simulink model "linear_system"  (R2023b)
settings: Solver=VariableStepAuto  StartTime=0.0  StopTime=60  RelTol=1e-3
values from neighbouring files (symbols this model uses):
  Alin = [0    -k/Jl + m*g*l*sin(x2_bar)/Jl                     0           k/Jl ... (first row only)    [collaborative_class_main.m]    (also in n0_collaborative_class_main.m = [ 0           -k/Jl + m*g*l*sin(x2_bar)/Jl             0    )
  Blin = [0; 0; 1/Jm; 0]    [collaborative_class_main.m]    (also in n0_collaborative_class_main.m)
  K = place(Alin, Blin, p)    [collaborative_class_main.m]    (also in n0_collaborative_class_main.m)
  K_H2_V = K_H2(:, 5)    [collaborative_class_main.m]    (also in n0_collaborative_class_main.m)
  K_H2_X = K_H2(:,1:4)    [collaborative_class_main.m]    (also in n0_collaborative_class_main.m)
  K_lq = R^(-1)*Blin'*P_lq    [n0_collaborative_class_main.m]
  K_lqeta = K_lqe(:, 5)    [collaborative_class_main.m]    (also in n0_collaborative_class_main.m = K_lq_ext(:,5))
  K_lqx = K_lqe(:,1:4)    [collaborative_class_main.m]    (also in n0_collaborative_class_main.m = K_lq_ext(:,1:4))
  Kv = -K_ext(1, 5)    [collaborative_class_main.m]    (also in n0_collaborative_class_main.m)
  Kx = -K_ext(1, 1:4)    [collaborative_class_main.m]    (also in n0_collaborative_class_main.m)
  x_bar = [x1_bar x2_bar x3_bar x4_bar]    [collaborative_class_main.m]    (also in n0_collaborative_class_main.m; svc_robot.m = [x1_bar x2_bar x3_bar x4_bar]')
settings Model: Creator=teoma  LastModifiedBy=alexandraspertini

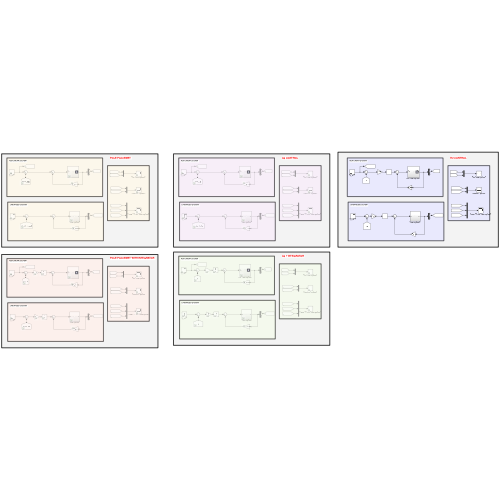
[thumbnail: Simulink's stored preview of the top-level diagram]
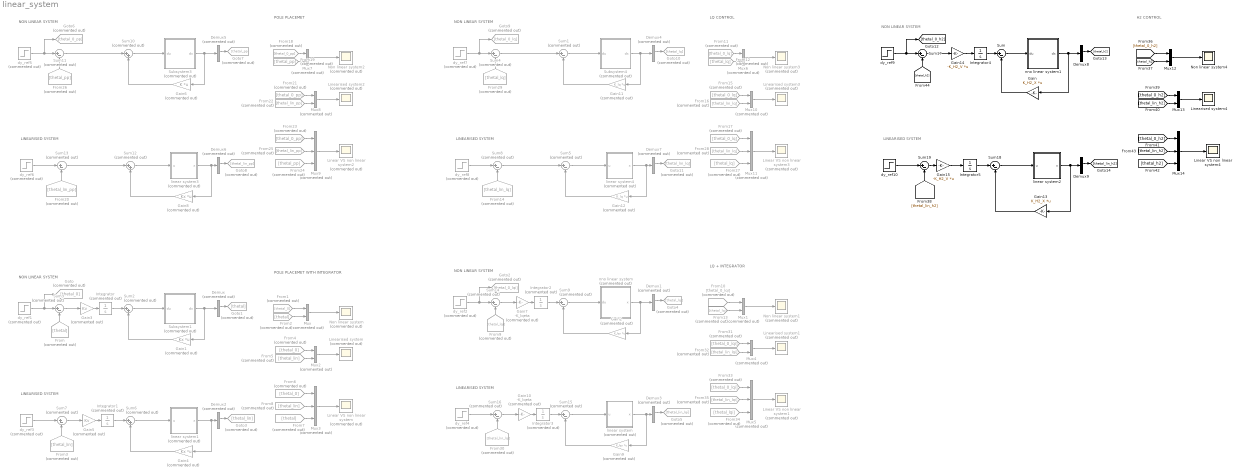
== system linear_system ==
  note: POLE PLACEMET WITH INTEGRATOR
  note: NON LINEAR SYSTEM
  note: LINEARISED SYSTEM
  note: POLE PLACEMET
  note: LINEARISED SYSTEM
  note: NON LINEAR SYSTEM
  note: NON LINEAR SYSTEM
  note: LQ CONTROL
  note: LINEARISED SYSTEM
  note: NON LINEAR SYSTEM
  note: LINEARISED SYSTEM
  note: LQ + INTEGRATOR
  note: LINEARISED SYSTEM
  note: H2 CONTROL
  note: NON LINEAR SYSTEM
  Demux{,1..7} (8 alike) : Demux  Commented=on
  Demux8 : Demux
  Demux9 : Demux
  From : From  Commented=on  GotoTag=thetal
  From1 : From  Commented=on  GotoTag=thetal_0
  From10 : From  Commented=on  GotoTag=thetal_0_lqi
  From11 : From  Commented=on  GotoTag=thetal_0_lq
  From12 : From  Commented=on  GotoTag=thetal_lq
  From13 : From  Commented=on  GotoTag=thetal_lqi
  From14 : From  Commented=on  GotoTag=thetal_lin_lq
  From15 : From  Commented=on  GotoTag=thetal_0_lq
  From16 : From  Commented=on  GotoTag=thetal_lin_lq
  From17 : From  Commented=on  GotoTag=thetal_0_lq
  From18 : From  Commented=on  GotoTag=thetal_0_pp
  From19 : From  Commented=on  GotoTag=thetal_pp
  From2 : From  Commented=on  GotoTag=thetal
  From20 : From  Commented=on  GotoTag=thetal_lin_pp
  From21 : From  Commented=on  GotoTag=thetal_0_pp
  From22 : From  Commented=on  GotoTag=thetal_lin_pp
  From23 : From  Commented=on  GotoTag=thetal_0_pp
  From24 : From  Commented=on  GotoTag=thetal_pp
  From25 : From  Commented=on  GotoTag=thetal_lin_pp
  From26 : From  Commented=on  GotoTag=thetal_pp
  From27 : From  Commented=on  GotoTag=thetal_lq
  From28 : From  Commented=on  GotoTag=thetal_lin_lq
  From29 : From  Commented=on  GotoTag=thetal_lq
  From3 : From  Commented=on  GotoTag=thetal_lin
  From30 : From  Commented=on  GotoTag=thetal_lin_lqi
  From31 : From  Commented=on  GotoTag=thetal_0_lqi
  From32 : From  Commented=on  GotoTag=thetal_lin_lqi
  From33 : From  Commented=on  GotoTag=thetal_0_lqi
  From34 : From  Commented=on  GotoTag=thetal_lqi
  From35 : From  Commented=on  GotoTag=thetal_lin_lqi
  From4 : From  Commented=on  GotoTag=thetal_0
  From5 : From  Commented=on  GotoTag=thetal_lin
  From6 : From  Commented=on  GotoTag=thetal_0
  From7 : From  Commented=on  GotoTag=thetal
  From8 : From  Commented=on  GotoTag=thetal_lin
  From9 : From  Commented=on  GotoTag=thetal_lqi
  Gain : Gain  Gain=K_H2_X  Multiplication=Matrix(K*u) (u vector)
  Gain1 : Gain  Commented=on  Gain=Kx  Multiplication=Matrix(K*u) (u vector)
  Gain10 : Gain  Commented=on  Gain=-K_lqeta
  Gain11 : Gain  Commented=on  Gain=K_lq  Multiplication=Matrix(K*u) (u vector)
  Gain12 : Gain  Commented=on  Gain=K_lq  Multiplication=Matrix(K*u) (u vector)
  Gain13 : Gain  Gain=K_H2_X  Multiplication=Matrix(K*u) (u vector)
  Gain14 : Gain  Gain=-K_H2_V  Multiplication=Matrix(K*u) (u vector)
  Gain15 : Gain  Gain=-K_H2_V  Multiplication=Matrix(K*u) (u vector)
  Gain2 : Gain  Commented=on  Gain=K_lqx  Multiplication=Matrix(K*u) (u vector)
  Gain3 : Gain  Commented=on  Gain=Kv
  Gain4 : Gain  Commented=on  Gain=Kx  Multiplication=Matrix(K*u) (u vector)
  Gain5 : Gain  Commented=on  Gain=Kv
  Gain6 : Gain  Commented=on  Gain=K  Multiplication=Matrix(K*u) (u vector)
  Gain7 : Gain  Commented=on  Gain=-K_lqeta
  Gain8 : Gain  Commented=on  Gain=Kx  Multiplication=Matrix(K*u) (u vector)
  Gain9 : Gain  Commented=on  Gain=K_lqx  Multiplication=Matrix(K*u) (u vector)
  Goto : Goto  Commented=on  GotoTag=thetal_0
  Goto1 : Goto  Commented=on  GotoTag=thetal
  Goto10 : Goto  Commented=on  GotoTag=thetal_lq
  Goto11 : Goto  Commented=on  GotoTag=thetal_lin_lq
  Goto2 : Goto  Commented=on  GotoTag=thetal_0_lqi
  Goto3 : Goto  Commented=on  GotoTag=thetal_lin
  Goto4 : Goto  Commented=on  GotoTag=thetal_lqi
  Goto5 : Goto  Commented=on  GotoTag=thetal_lin_lqi
  Goto6 : Goto  Commented=on  GotoTag=thetal_0_pp
  Goto7 : Goto  Commented=on  GotoTag=thetal_pp
  Goto8 : Goto  Commented=on  GotoTag=thetal_lin_pp
  Goto9 : Goto  Commented=on  GotoTag=thetal_0_lq
  Integrator{,1..3} (4 alike) : Integrator  Commented=on
  Integrator4 : Integrator
  Integrator5 : Integrator
  Linear VS non linear system{,1..3} (4 alike) : Scope  Commented=on
  Linear VS non linear system4 : Scope
  Linearised system{,1..3} (4 alike) : Scope  Commented=on
  Linearised system4 : Scope
  Mux{,1..2,4,6..8,10} (8 alike) : Mux  Commented=on  Inputs=2
  Mux{3,5,9,11} (4 alike) : Mux  Commented=on  Inputs=3
  Mux12 : Mux  Inputs=2
  Mux13 : Mux  Inputs=2
  Mux14 : Mux  Inputs=3
  Non linear system{,1..3} (4 alike) : Scope  Commented=on
  Non linear system4 : Scope
  Subsystem1 : Subsystem  Commented=on
  Subsystem3 : Subsystem  Commented=on
  Subsystem4 : Subsystem  Commented=on
  Sum{,17..19} (4 alike) : Sum  Inputs=|+-
  Sum{1,3..5,7..9,11,13..16} (12 alike) : Sum  Commented=on  Inputs=|+-
  Sum{2,6,10,12} (4 alike) : Sum  Commented=on  Inputs=|++
  dy_ref{1,3,5..6} (4 alike) : Step  Commented=on  After=pi/24  SampleTime=0
  dy_ref10 : Step  Time=0  After=pi/36  SampleTime=0
  dy_ref2 : Step  Commented=on  Time=0  After=pi/36  SampleTime=0
  dy_ref4 : Step  Commented=on  Time=0  After=pi/36  SampleTime=0
  dy_ref7 : Step  Commented=on  After=pi/36  SampleTime=0
  dy_ref8 : Step  Commented=on  After=pi/36  SampleTime=0
  dy_ref9 : Step  Time=0  After=pi/36  SampleTime=0
  linear system : Subsystem  Commented=on
  linear system1 : Subsystem  Commented=on
  linear system2 : Subsystem
  linear system3 : Subsystem  Commented=on
  linear system4 : Subsystem  Commented=on
  nno linear system : Subsystem  Commented=on
  nno linear system1 : Subsystem
  wires:
  Subsystem1/1(dx) -> Gain1/1, Demux/1
  Sum2/1 -> Subsystem1/1(du)
  Gain1/1 -> Sum2/2
  dy_ref1/1 -> Goto/1, Sum3/1
  Mux/1 -> Non linear system/1
  Sum3/1 -> Gain3/1
  Gain3/1 -> Integrator/1
  Integrator/1 -> Sum2/1
  Demux/2 -> Goto1/1
  From/1 -> Sum3/2
  From1/1 -> Mux/1
  From2/1 -> Mux/2
  dy_ref3/1 -> Sum7/1
  Sum7/1 -> Gain5/1
  Sum6/1 -> linear system1/1(u)
  From5/1 -> Mux2/2
  Gain4/1 -> Sum6/2
  Mux2/1 -> Linearised system/1
  Gain5/1 -> Integrator1/1
  Integrator1/1 -> Sum6/1
  From4/1 -> Mux2/1
  From3/1 -> Sum7/2
  Demux2/2 -> Goto3/1
  linear system1/1(x) -> Gain4/1, Demux2/1
  From6/1 -> Mux3/1
  From7/1 -> Mux3/3
  From8/1 -> Mux3/2
  Mux3/1 -> Linear VS non linear system/1
  Sum10/1 -> Subsystem3/1(du)
  Mux7/1 -> Non linear system2/1
  From21/1 -> Mux8/1
  From19/1 -> Mux7/2
  Gain6/1 -> Sum10/2
  Subsystem3/1(dx) -> Gain6/1, Demux5/1
  From23/1 -> Mux9/1
  Mux8/1 -> Linearised system2/1
  linear system3/1(x) -> Gain8/1, Demux6/1
  Demux5/2 -> Goto7/1
  From26/1 -> Sum11/2
  From18/1 -> Mux7/1
  Gain8/1 -> Sum12/2
  Demux6/2 -> Goto8/1
  From20/1 -> Sum13/2
  Mux9/1 -> Linear VS non linear system2/1
  dy_ref6/1 -> Sum13/1
  From22/1 -> Mux8/2
  From25/1 -> Mux9/2
  Sum12/1 -> linear system3/1(u)
  From24/1 -> Mux9/3
  dy_ref5/1 -> Goto6/1, Sum11/1
  Sum11/1 -> Sum10/1
  Sum13/1 -> Sum12/1
  From33/1 -> Mux5/1
  Sum8/1 -> Sum5/1
  From29/1 -> Sum4/2
  Subsystem4/1(dx) -> Gain11/1, Demux4/1
  Integrator3/1 -> Sum15/1
  From17/1 -> Mux11/1
  Sum1/1 -> Subsystem4/1(du)
  Mux1/1 -> Non linear system1/1
  From32/1 -> Mux4/2
  Mux10/1 -> Linearised system3/1
  Demux3/2 -> Goto5/1
  Demux7/2 -> Goto11/1
  From15/1 -> Mux10/1
  Demux1/2 -> Goto4/1
  Mux6/1 -> Non linear system3/1
  From14/1 -> Sum8/2
  From11/1 -> Mux6/1
  From27/1 -> Mux11/3
  Sum4/1 -> Sum1/1
  From31/1 -> Mux4/1
  Gain11/1 -> Sum1/2
  Sum15/1 -> linear system/1(u)
  dy_ref2/1 -> Goto2/1, Sum14/1
  Gain7/1 -> Integrator2/1
  Gain2/1 -> Sum9/2
  From10/1 -> Mux1/1
  From12/1 -> Mux6/2
  Gain9/1 -> Sum15/2
  dy_ref4/1 -> Sum16/1
  nno linear system/1(x) -> Gain2/1, Demux1/1
  From35/1 -> Mux5/2
  Gain10/1 -> Integrator3/1
  Sum16/1 -> Gain10/1
  Sum5/1 -> linear system4/1(u)
  From9/1 -> Sum14/2
  dy_ref8/1 -> Sum8/1
  From13/1 -> Mux1/2
  linear system/1(x) -> Gain9/1, Demux3/1
  Sum14/1 -> Gain7/1
  dy_ref7/1 -> Goto9/1, Sum4/1
  Mux4/1 -> Linearised system1/1
  Mux11/1 -> Linear VS non linear system3/1
  linear system4/1(x) -> Gain12/1, Demux7/1
  From16/1 -> Mux10/2
  From28/1 -> Mux11/2
  Sum9/1 -> nno linear system/1(du)
  Mux5/1 -> Linear VS non linear system1/1
  Demux4/2 -> Goto10/1
  From30/1 -> Sum16/2
  Gain12/1 -> Sum5/2
  From34/1 -> Mux5/3
  Integrator2/1 -> Sum9/1
  [thetal_lin_h2] -> Mux13/2
  Demux9/2 -> [thetal_lin_h2]
  [thetal_lin_h2] -> Mux14/2
  [thetal_lin_h2] -> Sum19/2
  [thetal_h2] -> Mux12/2
  Mux12/1 -> Non linear system4/1
  [thetal_h2] -> Sum17/2
  [thetal_h2] -> Mux14/3
  dy_ref10/1 -> Sum19/1
  [thetal_0_h2] -> Mux12/1
  Demux8/2 -> [thetal_h2]
  [thetal_0_h2] -> Mux13/1
  nno linear system1/1(dx) -> Gain/1, Demux8/1
  dy_ref9/1 -> [thetal_0_h2], Sum17/1
  [thetal_0_h2] -> Mux14/1
  Mux14/1 -> Linear VS non linear system4/1
  linear system2/1(x) -> Gain13/1, Demux9/1
  Mux13/1 -> Linearised system4/1
  Gain/1 -> Sum/2
  Sum/1 -> nno linear system1/1(du)
  Sum18/1 -> linear system2/1(u)
  Gain13/1 -> Sum18/2
  Gain14/1 -> Integrator4/1
  Gain15/1 -> Integrator5/1
  Sum17/1 -> Gain14/1
  Integrator4/1 -> Sum/1
  Sum19/1 -> Gain15/1
  Integrator5/1 -> Sum18/1

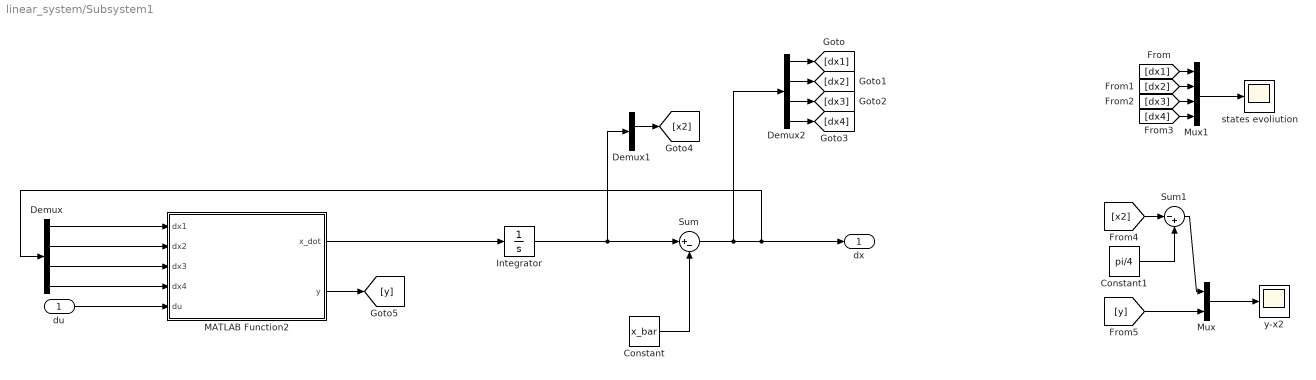
== system linear_system/Subsystem1 ==
  du : Inport
  Constant : Constant  Value=x_bar
  Constant1 : Constant  Value=pi/4
  Demux : Demux
  Demux1 : Demux
  Demux2 : Demux
  Integrator : Integrator  InitialCondition=0.001
  MATLAB Function2 : MATLAB Function  TreatAsAtomicUnit=on
  Mux : Mux  Inputs=2
  Mux1 : Mux
  Sum : Sum  Inputs=|+-
  Sum1 : Sum  Inputs=|-+
  "states evoliution " : Scope
  y-x2 : Scope
  dx : Outport
  wires:
  du/1 -> MATLAB Function2/5(du)
  MATLAB Function2/2(y) -> [y]
  Demux/1 -> MATLAB Function2/1(dx1)
  Demux/2 -> MATLAB Function2/2(dx2)
  Demux/3 -> MATLAB Function2/3(dx3)
  Demux/4 -> MATLAB Function2/4(dx4)
  Constant/1 -> Sum/2
  MATLAB Function2/1(x_dot) -> Integrator/1
  Integrator/1 -> Demux1/1, Sum/1
  Sum/1 -> Demux2/1, dx/1, Demux/1
  Mux/1 -> y-x2/1
  Sum1/1 -> Mux/1
  Constant1/1 -> Sum1/2
  Demux2/1 -> [dx1]
  Demux2/2 -> [dx2]
  Demux2/3 -> [dx3]
  Demux2/4 -> [dx4]
  [dx1] -> Mux1/1
  [dx2] -> Mux1/2
  [dx3] -> Mux1/3
  [dx4] -> Mux1/4
  Mux1/1 -> "states evoliution "/1
  Demux1/2 -> [x2]
  [x2] -> Sum1/1
  [y] -> Mux/2

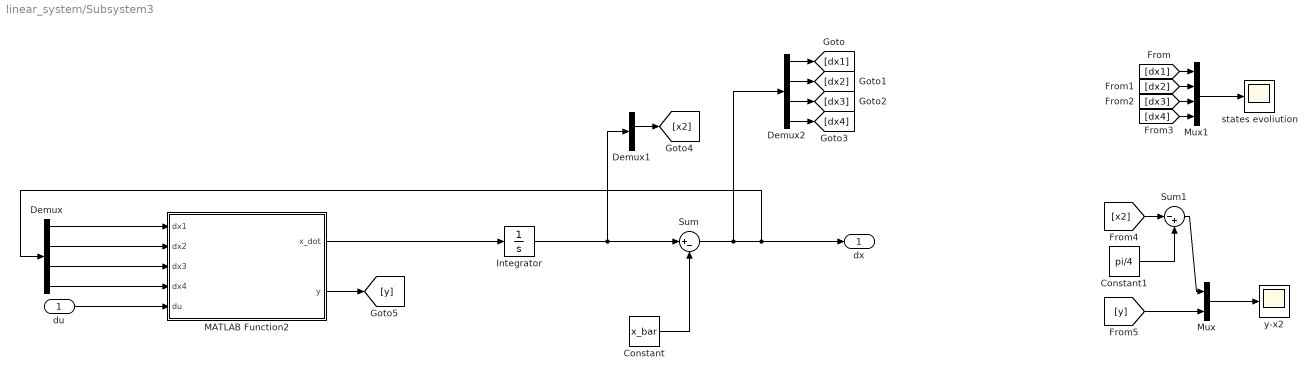
== system linear_system/Subsystem3 ==
  du : Inport
  Constant : Constant  Value=x_bar
  Constant1 : Constant  Value=pi/4
  Demux : Demux
  Demux1 : Demux
  Demux2 : Demux
  Integrator : Integrator  InitialCondition=0.001
  MATLAB Function2 : MATLAB Function  TreatAsAtomicUnit=on
  Mux : Mux  Inputs=2
  Mux1 : Mux
  Sum : Sum  Inputs=|+-
  Sum1 : Sum  Inputs=|-+
  "states evoliution " : Scope
  y-x2 : Scope
  dx : Outport
  wires:
  du/1 -> MATLAB Function2/5(du)
  MATLAB Function2/2(y) -> [y]
  Demux/1 -> MATLAB Function2/1(dx1)
  Demux/2 -> MATLAB Function2/2(dx2)
  Demux/3 -> MATLAB Function2/3(dx3)
  Demux/4 -> MATLAB Function2/4(dx4)
  Constant/1 -> Sum/2
  MATLAB Function2/1(x_dot) -> Integrator/1
  Integrator/1 -> Demux1/1, Sum/1
  Sum/1 -> Demux2/1, dx/1, Demux/1
  Mux/1 -> y-x2/1
  Sum1/1 -> Mux/1
  Constant1/1 -> Sum1/2
  Demux2/1 -> [dx1]
  Demux2/2 -> [dx2]
  Demux2/3 -> [dx3]
  Demux2/4 -> [dx4]
  [dx1] -> Mux1/1
  [dx2] -> Mux1/2
  [dx3] -> Mux1/3
  [dx4] -> Mux1/4
  Mux1/1 -> "states evoliution "/1
  Demux1/2 -> [x2]
  [x2] -> Sum1/1
  [y] -> Mux/2

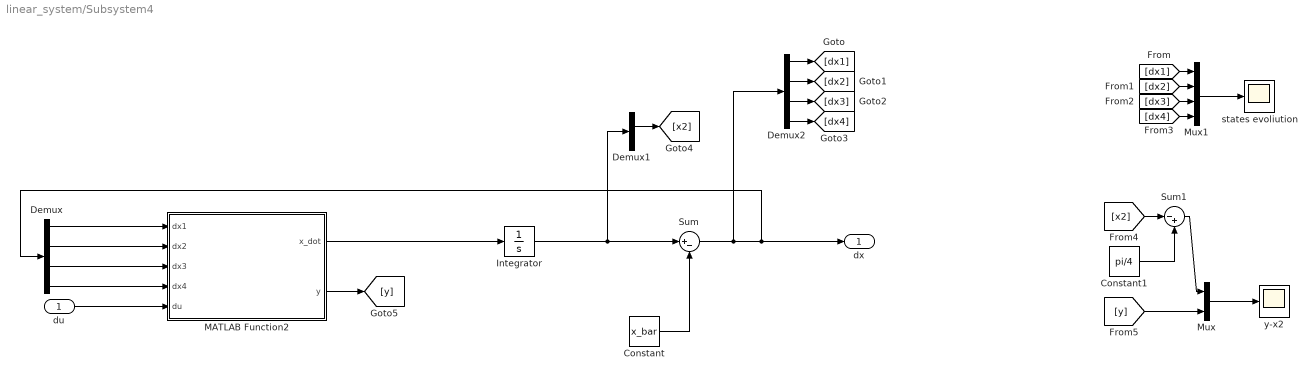
== system linear_system/Subsystem4 ==
  du : Inport
  Constant : Constant  Value=x_bar
  Constant1 : Constant  Value=pi/4
  Demux : Demux
  Demux1 : Demux
  Demux2 : Demux
  Integrator : Integrator  InitialCondition=0.001
  MATLAB Function2 : MATLAB Function  TreatAsAtomicUnit=on
  Mux : Mux  Inputs=2
  Mux1 : Mux
  Sum : Sum  Inputs=|+-
  Sum1 : Sum  Inputs=|-+
  "states evoliution " : Scope
  y-x2 : Scope
  dx : Outport
  wires:
  du/1 -> MATLAB Function2/5(du)
  MATLAB Function2/2(y) -> [y]
  Demux/1 -> MATLAB Function2/1(dx1)
  Demux/2 -> MATLAB Function2/2(dx2)
  Demux/3 -> MATLAB Function2/3(dx3)
  Demux/4 -> MATLAB Function2/4(dx4)
  Constant/1 -> Sum/2
  MATLAB Function2/1(x_dot) -> Integrator/1
  Integrator/1 -> Demux1/1, Sum/1
  Sum/1 -> Demux2/1, dx/1, Demux/1
  Mux/1 -> y-x2/1
  Sum1/1 -> Mux/1
  Constant1/1 -> Sum1/2
  Demux2/1 -> [dx1]
  Demux2/2 -> [dx2]
  Demux2/3 -> [dx3]
  Demux2/4 -> [dx4]
  [dx1] -> Mux1/1
  [dx2] -> Mux1/2
  [dx3] -> Mux1/3
  [dx4] -> Mux1/4
  Mux1/1 -> "states evoliution "/1
  Demux1/2 -> [x2]
  [x2] -> Sum1/1
  [y] -> Mux/2

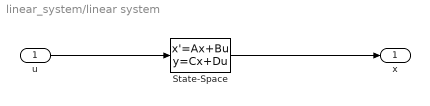
== system linear_system/linear system ==
  u : Inport
  State-Space : StateSpace  A=Alin  B=Blin  C=eye(4)  D=zeros(4,1)  InitialCondition=0
  x : Outport
  wires:
  State-Space/1 -> x/1
  u/1 -> State-Space/1

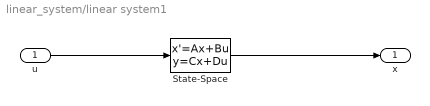
== system linear_system/linear system1 ==
  u : Inport
  State-Space : StateSpace  A=Alin  B=Blin  C=eye(4)  D=zeros(4,1)  InitialCondition=0
  x : Outport
  wires:
  State-Space/1 -> x/1
  u/1 -> State-Space/1

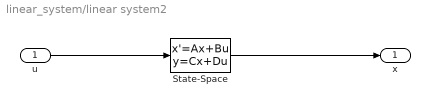
== system linear_system/linear system2 ==
  u : Inport
  State-Space : StateSpace  A=Alin  B=Blin  C=eye(4)  D=zeros(4,1)  InitialCondition=0
  x : Outport
  wires:
  State-Space/1 -> x/1
  u/1 -> State-Space/1

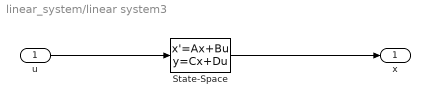
== system linear_system/linear system3 ==
  u : Inport
  State-Space : StateSpace  A=Alin  B=Blin  C=eye(4)  D=zeros(4,1)  InitialCondition=0
  x : Outport
  wires:
  State-Space/1 -> x/1
  u/1 -> State-Space/1

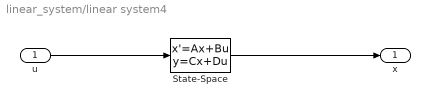
== system linear_system/linear system4 ==
  u : Inport
  State-Space : StateSpace  A=Alin  B=Blin  C=eye(4)  D=zeros(4,1)  InitialCondition=0
  x : Outport
  wires:
  State-Space/1 -> x/1
  u/1 -> State-Space/1

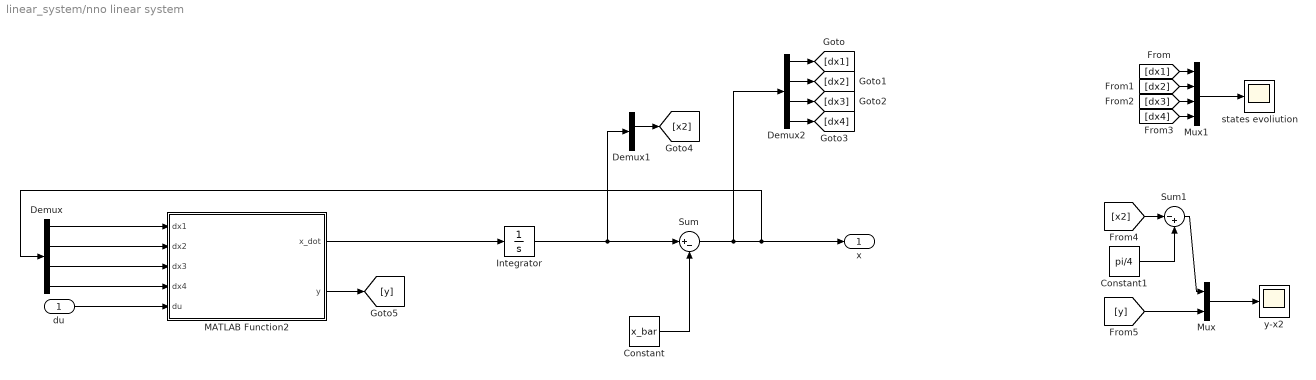
== system linear_system/nno linear system ==
  du : Inport
  Constant : Constant  Value=x_bar
  Constant1 : Constant  Value=pi/4
  Demux : Demux
  Demux1 : Demux
  Demux2 : Demux
  Integrator : Integrator  InitialCondition=0.001
  MATLAB Function2 : MATLAB Function  TreatAsAtomicUnit=on
  Mux : Mux  Inputs=2
  Mux1 : Mux
  Sum : Sum  Inputs=|+-
  Sum1 : Sum  Inputs=|-+
  "states evoliution " : Scope
  y-x2 : Scope
  x : Outport
  wires:
  du/1 -> MATLAB Function2/5(du)
  MATLAB Function2/2(y) -> [y]
  Demux/1 -> MATLAB Function2/1(dx1)
  Demux/2 -> MATLAB Function2/2(dx2)
  Demux/3 -> MATLAB Function2/3(dx3)
  Demux/4 -> MATLAB Function2/4(dx4)
  Constant/1 -> Sum/2
  MATLAB Function2/1(x_dot) -> Integrator/1
  Integrator/1 -> Demux1/1, Sum/1
  Sum/1 -> Demux2/1, x/1, Demux/1
  Mux/1 -> y-x2/1
  Sum1/1 -> Mux/1
  Constant1/1 -> Sum1/2
  Demux2/1 -> [dx1]
  Demux2/2 -> [dx2]
  Demux2/3 -> [dx3]
  Demux2/4 -> [dx4]
  [dx1] -> Mux1/1
  [dx2] -> Mux1/2
  [dx3] -> Mux1/3
  [dx4] -> Mux1/4
  Mux1/1 -> "states evoliution "/1
  Demux1/2 -> [x2]
  [x2] -> Sum1/1
  [y] -> Mux/2

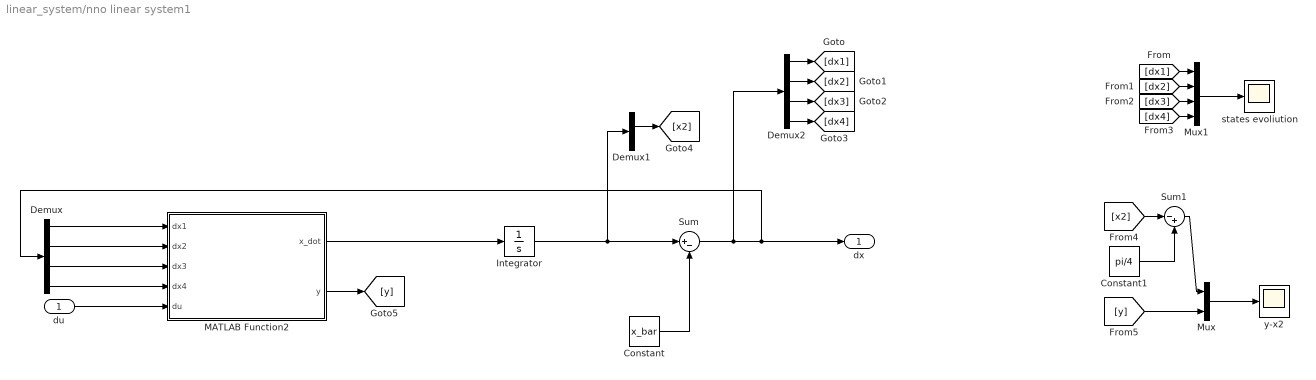
== system linear_system/nno linear system1 ==
  du : Inport
  Constant : Constant  Value=x_bar
  Constant1 : Constant  Value=pi/4
  Demux : Demux
  Demux1 : Demux
  Demux2 : Demux
  Integrator : Integrator  InitialCondition=0.001
  MATLAB Function2 : MATLAB Function  TreatAsAtomicUnit=on
  Mux : Mux  Inputs=2
  Mux1 : Mux
  Sum : Sum  Inputs=|+-
  Sum1 : Sum  Inputs=|-+
  "states evoliution " : Scope
  y-x2 : Scope
  dx : Outport
  wires:
  du/1 -> MATLAB Function2/5(du)
  MATLAB Function2/2(y) -> [y]
  Demux/1 -> MATLAB Function2/1(dx1)
  Demux/2 -> MATLAB Function2/2(dx2)
  Demux/3 -> MATLAB Function2/3(dx3)
  Demux/4 -> MATLAB Function2/4(dx4)
  Constant/1 -> Sum/2
  MATLAB Function2/1(x_dot) -> Integrator/1
  Integrator/1 -> Demux1/1, Sum/1
  Sum/1 -> Demux2/1, dx/1, Demux/1
  Mux/1 -> y-x2/1
  Sum1/1 -> Mux/1
  Constant1/1 -> Sum1/2
  Demux2/1 -> [dx1]
  Demux2/2 -> [dx2]
  Demux2/3 -> [dx3]
  Demux2/4 -> [dx4]
  [dx1] -> Mux1/1
  [dx2] -> Mux1/2
  [dx3] -> Mux1/3
  [dx4] -> Mux1/4
  Mux1/1 -> "states evoliution "/1
  Demux1/2 -> [x2]
  [x2] -> Sum1/1
  [y] -> Mux/2

== matlab function linear_system/nno linear system/MATLAB Function2 ==
  data: dx1 input; dx2 input; dx3 input; dx4 input; du input; x_dot output; y output
function [x_dot, y]  = fcn(dx1,dx2,dx3,dx4, du)

k = 0.8;
Jm = 4e-4;
Jl= 4e-4;
Bm = 0.015;
Bl = 0;
m = 0.3;
l = 0.3;
g = 9.81;
x1_bar = 0;
x2_bar = pi/4;
x3_bar = 0;
x4_bar = m*g*l*cos(x2_bar)/k + x2_bar;
u_bar= m*g*l*cos(x2_bar);


x1_dot = -k/Jl*(dx2+x2_bar)-m*g*l/Jl*(cos(dx2+x2_bar))+k/Jl*(dx4+x4_bar);
x2_dot = dx1+x1_bar;
x3_dot = k/Jm*(dx2+x2_bar)-Bm/Jm*(dx3+x3_bar)-k/Jm*(dx4+x4_bar)+1/Jm*(du+u_bar);
x4_dot = dx3+x3_bar;
y = pi/4 - (dx2+x2_bar);

x_dot = zeros(1,4);
x_dot(1) = x1_dot;
x_dot(2) = x2_dot;
x_dot(3) = x3_dot;
x_dot(4) = x4_dot;

== matlab function linear_system/Subsystem3/MATLAB Function2 ==
  data: dx1 input; dx2 input; dx3 input; dx4 input; du input; x_dot output; y output
function [x_dot, y]  = fcn(dx1,dx2,dx3,dx4, du)

k = 0.8;
Jm = 4e-4;
Jl= 4e-4;
Bm = 0.015;
Bl = 0;
m = 0.3;
l = 0.3;
g = 9.81;
x1_bar = 0;
x2_bar = pi/4;
x3_bar = 0;
x4_bar = m*g*l*cos(x2_bar)/k + x2_bar;
u_bar= m*g*l*cos(x2_bar);


x1_dot = -k/Jl*(dx2+x2_bar)-m*g*l/Jl*(cos(dx2+x2_bar))+k/Jl*(dx4+x4_bar);
x2_dot = dx1+x1_bar;
x3_dot = k/Jm*(dx2+x2_bar)-Bm/Jm*(dx3+x3_bar)-k/Jm*(dx4+x4_bar)+1/Jm*(du+u_bar);
x4_dot = dx3+x3_bar;
y = pi/4 - (dx2+x2_bar);

x_dot = zeros(1,4);
x_dot(1) = x1_dot;
x_dot(2) = x2_dot;
x_dot(3) = x3_dot;
x_dot(4) = x4_dot;

== matlab function linear_system/Subsystem4/MATLAB Function2 ==
  data: dx1 input; dx2 input; dx3 input; dx4 input; du input; x_dot output; y output
function [x_dot, y]  = fcn(dx1,dx2,dx3,dx4, du)

k = 0.8;
Jm = 4e-4;
Jl= 4e-4;
Bm = 0.015;
Bl = 0;
m = 0.3;
l = 0.3;
g = 9.81;
x1_bar = 0;
x2_bar = pi/4;
x3_bar = 0;
x4_bar = m*g*l*cos(x2_bar)/k + x2_bar;
u_bar= m*g*l*cos(x2_bar);


x1_dot = -k/Jl*(dx2+x2_bar)-m*g*l/Jl*(cos(dx2+x2_bar))+k/Jl*(dx4+x4_bar);
x2_dot = dx1+x1_bar;
x3_dot = k/Jm*(dx2+x2_bar)-Bm/Jm*(dx3+x3_bar)-k/Jm*(dx4+x4_bar)+1/Jm*(du+u_bar);
x4_dot = dx3+x3_bar;
y = pi/4 - (dx2+x2_bar);

x_dot = zeros(1,4);
x_dot(1) = x1_dot;
x_dot(2) = x2_dot;
x_dot(3) = x3_dot;
x_dot(4) = x4_dot;

== matlab function linear_system/Subsystem1/MATLAB Function2 ==
  data: dx1 input; dx2 input; dx3 input; dx4 input; du input; x_dot output; y output
function [x_dot, y]  = fcn(dx1,dx2,dx3,dx4, du)

k = 0.8;
Jm = 4e-4;
Jl= 4e-4;
Bm = 0.015;
Bl = 0;
m = 0.3;
l = 0.3;
g = 9.81;
x1_bar = 0;
x2_bar = pi/4;
x3_bar = 0;
x4_bar = m*g*l*cos(x2_bar)/k + x2_bar;
u_bar= m*g*l*cos(x2_bar);


x1_dot = -k/Jl*(dx2+x2_bar)-m*g*l/Jl*(cos(dx2+x2_bar))+k/Jl*(dx4+x4_bar);
x2_dot = dx1+x1_bar;
x3_dot = k/Jm*(dx2+x2_bar)-Bm/Jm*(dx3+x3_bar)-k/Jm*(dx4+x4_bar)+1/Jm*(du+u_bar);
x4_dot = dx3+x3_bar;
y = pi/4 - (dx2+x2_bar);

x_dot = zeros(1,4);
x_dot(1) = x1_dot;
x_dot(2) = x2_dot;
x_dot(3) = x3_dot;
x_dot(4) = x4_dot;

== matlab function linear_system/nno linear system1/MATLAB Function2 ==
  data: dx1 input; dx2 input; dx3 input; dx4 input; du input; x_dot output; y output
function [x_dot, y]  = fcn(dx1,dx2,dx3,dx4, du)

k = 0.8;
Jm = 4e-4;
Jl= 4e-4;
Bm = 0.015;
Bl = 0;
m = 0.3;
l = 0.3;
g = 9.81;
x1_bar = 0;
x2_bar = pi/4;
x3_bar = 0;
x4_bar = m*g*l*cos(x2_bar)/k + x2_bar;
u_bar= m*g*l*cos(x2_bar);


x1_dot = -k/Jl*(dx2+x2_bar)-m*g*l/Jl*(cos(dx2+x2_bar))+k/Jl*(dx4+x4_bar);
x2_dot = dx1+x1_bar;
x3_dot = k/Jm*(dx2+x2_bar)-Bm/Jm*(dx3+x3_bar)-k/Jm*(dx4+x4_bar)+1/Jm*(du+u_bar);
x4_dot = dx3+x3_bar;
y = pi/4 - (dx2+x2_bar);

x_dot = zeros(1,4);
x_dot(1) = x1_dot;
x_dot(2) = x2_dot;
x_dot(3) = x3_dot;
x_dot(4) = x4_dot;
